simulink model "qbot2_sim_2019b"  (R2019b)
settings: Solver=FixedStepAuto  StartTime=0.0  StopTime=P.t_end  FixedStep=P.dt  RelTol=1e-3
InitFcn:
  | % load_qbot2_sim
StopFcn:
  | if (P.plotsim_flag)
  |     plot_sim(out, P)
  | end
(part 1 of 2)
settings Model: Creator=David L Olson  LastModifiedBy=divad

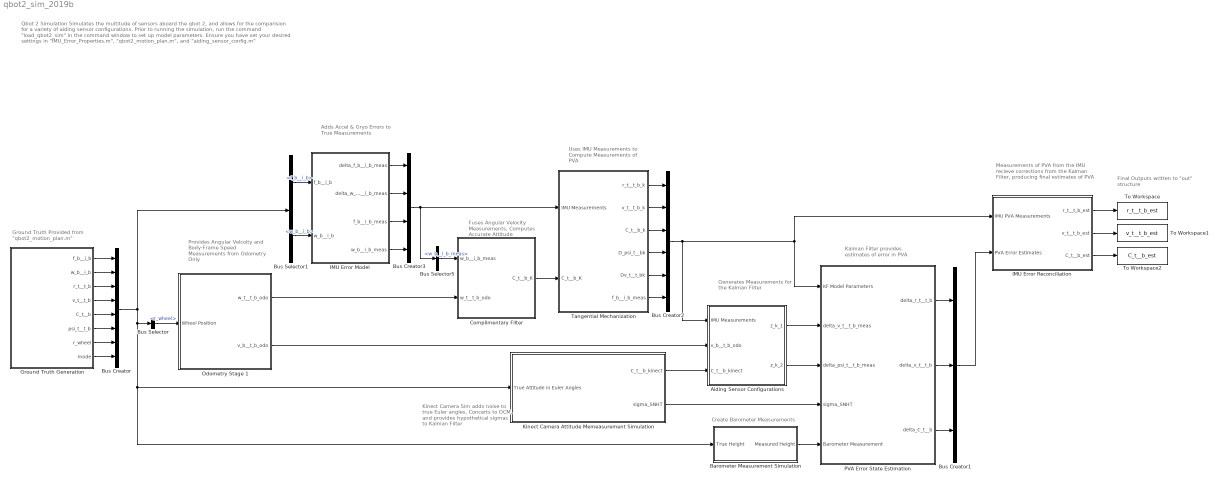
== system qbot2_sim_2019b ==
  note: Final Outputs written to "out" structure
  note: Create Barometer Measurements
  note: Qbot 2 Simulation
      |
      | Simulates the multitude of sensors aboard the qbot 2, and allows for the comparision for a variety of aiding sensor configurations.
      |
      | Prior to running the simulation, run the command "load_qbot2_sim" in the command window to set up model parameters.
      | Ensure you have set your desired settings in "IMU_Error_Properties.m", "qbot2_motion_plan.m", and "aiding_sensor_config.m"
  note: Measurements of PVA from the IMU recieve corrections from the Kalman Filter, producing final estimates of PVA
  note: Kalman Filter provides estimates of error in PVA
  note: Generates Measurements for the Kalman Filter
  note: Kinect Camera Sim adds noise to true Euler angles, Concerts to DCM, and provides hypothetical sigmas to Kalman Filter
  note: Uses IMU Measurements to Compute Measurements of PVA
  note: Fuses Angular Velocity Measurements, Computes Accurate Attitude
  note: Adds Accel & Gryo Errors to True Measurements
  note: Provides Angular Velcoity and Body-Frame Speed Measurements from Odometry Only
  note: Ground Truth Provided from "qbot2_motion_plan.m"
  Aiding Sensor Configurations : Subsystem
  Barometer Measurement Simulation : Subsystem
  Bus Creator : BusCreator  Inputs=8
  Bus Creator1 : BusCreator  Inputs=3
  Bus Creator2 : BusCreator  Inputs=6
  Bus Creator3 : BusCreator  Inputs=4
  Bus Selector : BusSelector  OutputSignals=r_wheel
  Bus Selector1 : BusSelector  OutputSignals=f_b__i_b,w_b__i_b
  Bus Selector5 : BusSelector  OutputSignals=w_b__i_b_meas
  Complimentary Filter : Subsystem
  Ground Truth Generation : Subsystem
  IMU Error Model : Subsystem
  IMU Error Reconciliation : Subsystem
  Kinect Camera Attitude Memeasurement Simulation : Subsystem
  Odometry Stage 1 : Subsystem
  PVA Error State Estimation : Subsystem
  Tangential Mechanization : Subsystem
  To Workspace : ToWorkspace  VariableName=r_t__t_b_est  SampleTime=-1
  To Workspace1 : ToWorkspace  VariableName=v_t__t_b_est  SampleTime=-1
  To Workspace2 : ToWorkspace  VariableName=C_t__b_est  SampleTime=-1
  wires:
  Ground Truth Generation/1(f_b__i_b) -> Bus Creator/1
  Ground Truth Generation/2(w_b__i_b) -> Bus Creator/2
  Ground Truth Generation/3(r_t__t_b) -> Bus Creator/3
  Ground Truth Generation/4(v_t__t_b) -> Bus Creator/4
  Ground Truth Generation/5(C_t__b) -> Bus Creator/5
  Bus Creator/1 -> Bus Selector1/1, Barometer Measurement Simulation/1(True Height), Kinect Camera Attitude Memeasurement Simulation/1(True Attitude in Euler Angles), Bus Selector/1
  Bus Selector/1 -> Odometry Stage 1/1(Wheel Position)  "<r_wheel>"
  Odometry Stage 1/1(w_t__t_b_odo) -> Complimentary Filter/2("w_t__t_b_odo ")
  Odometry Stage 1/2(v_b__t_b_odo) -> Aiding Sensor Configurations/2(v_b__t_b_odo)
  Aiding Sensor Configurations/1(z_k_1) -> PVA Error State Estimation/2(delta_v_t__t_b_meas)
  Aiding Sensor Configurations/2(z_k_2) -> PVA Error State Estimation/3(delta_psi_t__t_b_meas)
  Ground Truth Generation/6(psi_t__t_b) -> Bus Creator/6
  Ground Truth Generation/7(r_wheel) -> Bus Creator/7
  Ground Truth Generation/8(mode) -> Bus Creator/8
  Bus Selector1/1 -> IMU Error Model/1(f_b__i_b)  "<f_b__i_b>"
  Bus Selector1/2 -> IMU Error Model/2(w_b__i_b)  "<w_b__i_b>"
  Complimentary Filter/1(C_t__b_K) -> Tangential Mechanization/2("C_t__b_K ")
  Tangential Mechanization/1(r_t__t_b_k) -> Bus Creator2/1
  Tangential Mechanization/2(v_t__t_b_k) -> Bus Creator2/2
  Tangential Mechanization/3(C_t__b_k) -> Bus Creator2/3
  IMU Error Model/1(delta_f_b__i_b_meas) -> Bus Creator3/1
  IMU Error Model/2(delta_w_b__i_b_meas) -> Bus Creator3/2
  IMU Error Model/3(f_b__i_b_meas) -> Bus Creator3/3
  IMU Error Model/4(w_b__i_b_meas) -> Bus Creator3/4
  Bus Selector5/1 -> Complimentary Filter/1(w_b__i_b_meas)  "<w_b__i_b_meas>"
  Bus Creator3/1 -> Tangential Mechanization/1(IMU Measurements), Bus Selector5/1
  Tangential Mechanization/4(D_psi_t__bk) -> Bus Creator2/4
  Tangential Mechanization/5(Dv_t__t_bk) -> Bus Creator2/5
  Bus Creator2/1 -> IMU Error Reconciliation/1(IMU PVA Measurements), PVA Error State Estimation/1(KF Model Parameters), Aiding Sensor Configurations/1(IMU Measurements)
  Tangential Mechanization/6(f_b__i_b_meas) -> Bus Creator2/6
  PVA Error State Estimation/1(delta_r_t__t_b) -> Bus Creator1/1
  PVA Error State Estimation/2(delta_v_t__t_b) -> Bus Creator1/2
  PVA Error State Estimation/3(delta_C_t__b) -> Bus Creator1/3
  Barometer Measurement Simulation/1(Measured Height) -> PVA Error State Estimation/5(Barometer Measurement)
  Bus Creator1/1 -> IMU Error Reconciliation/2(PVA Error Estimates)
  IMU Error Reconciliation/1(r_t__t_b_est) -> To Workspace/1
  IMU Error Reconciliation/2(v_t__t_b_est) -> To Workspace1/1
  IMU Error Reconciliation/3(C_t__b_est) -> To Workspace2/1
  Kinect Camera Attitude Memeasurement Simulation/1(C_t__b_kinect) -> Aiding Sensor Configurations/3(C_t__b_kinect)
  Kinect Camera Attitude Memeasurement Simulation/2(sigma_SNHT) -> PVA Error State Estimation/4(sigma_SNHT)

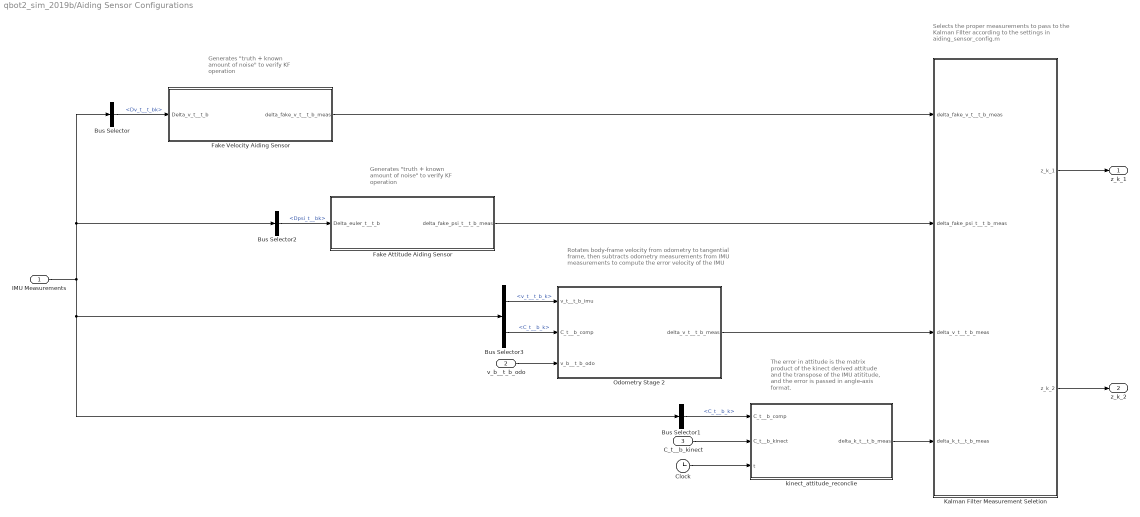
== system qbot2_sim_2019b/Aiding Sensor Configurations ==
  note: Selects the proper measurements to pass to the Kalman FIlter according to the settings in aiding_sensor_config.m
  note: The error in attitude is the matrix product of the kinect derived attitude and the transpose of the IMU atititude, and the error is passed in angle-axis format.
  note: Rotates body-frame velocity from odometry to tangential frame, then subtracts odometry measurements from IMU measurements to compute the error velocity of the IMU
  note: Generates "truth + known amount of noise" to verify KF operation
  note: Generates "truth + known amount of noise" to verify KF operation
  IMU Measurements : Inport
  v_b__t_b_odo : Inport  Port=2
  C_t__b_kinect : Inport  Port=3
  Bus Selector : BusSelector  OutputSignals=Dv_t__t_bk
  Bus Selector1 : BusSelector  OutputSignals=C_t__b_k
  Bus Selector2 : BusSelector  OutputSignals=Dpsi_t__bk
  Bus Selector3 : BusSelector  OutputSignals=v_t__t_b_k,C_t__b_k
  Clock : Clock
  Fake Attitude Aiding Sensor : MATLAB Function  TreatAsAtomicUnit=on
  Fake Velocity Aiding Sensor : MATLAB Function  TreatAsAtomicUnit=on
  Kalman Filter Measurement Seletion : MATLAB Function  TreatAsAtomicUnit=on
  Odometry Stage 2 : Subsystem
  kinect_attitude_reconclie : MATLAB Function  TreatAsAtomicUnit=on
  z_k_1 : Outport
  z_k_2 : Outport  Port=2
  wires:
  v_b__t_b_odo/1 -> Odometry Stage 2/3(v_b__t_b_odo)
  Fake Attitude Aiding Sensor/1(delta_fake_psi_t__t_b_meas) -> Kalman Filter Measurement Seletion/2(delta_fake_psi_t__t_b_meas)
  Fake Velocity Aiding Sensor/1(delta_fake_v_t__t_b_meas) -> Kalman Filter Measurement Seletion/1(delta_fake_v_t__t_b_meas)
  Odometry Stage 2/1(delta_v_t__t_b_meas) -> Kalman Filter Measurement Seletion/3(delta_v_t__t_b_meas)
  Kalman Filter Measurement Seletion/1(z_k_1) -> z_k_1/1
  Kalman Filter Measurement Seletion/2(z_k_2) -> z_k_2/1
  Bus Selector1/1 -> kinect_attitude_reconclie/1(C_t__b_comp)  "<C_t__b_k>"
  C_t__b_kinect/1 -> kinect_attitude_reconclie/2(C_t__b_kinect)
  kinect_attitude_reconclie/1(delta_k_t__t_b_meas) -> Kalman Filter Measurement Seletion/4(delta_k_t__t_b_meas)
  Bus Selector/1 -> Fake Velocity Aiding Sensor/1(Delta_v_t__t_b)  "<Dv_t__t_bk>"
  Bus Selector2/1 -> Fake Attitude Aiding Sensor/1(Delta_euler_t__t_b)  "<Dpsi_t__bk>"
  Bus Selector3/1 -> Odometry Stage 2/1(v_t__t_b_imu)  "<v_t__t_b_k>"
  Bus Selector3/2 -> Odometry Stage 2/2(C_t__b_comp)  "<C_t__b_k>"
  IMU Measurements/1 -> Bus Selector3/1, Bus Selector1/1, Bus Selector/1, Bus Selector2/1
  Clock/1 -> kinect_attitude_reconclie/3(t)

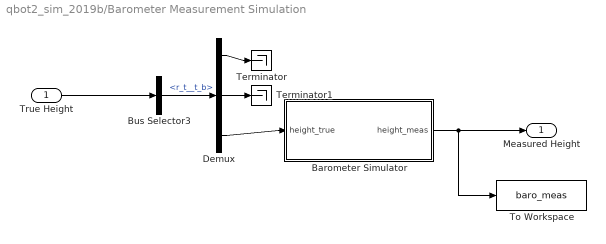
== system qbot2_sim_2019b/Barometer Measurement Simulation ==
  True Height : Inport
  Barometer Simulator : MATLAB Function  TreatAsAtomicUnit=on
  Bus Selector3 : BusSelector  OutputSignals=r_t__t_b
  Demux : Demux  Outputs=3
  Terminator : Terminator
  Terminator1 : Terminator
  To Workspace : ToWorkspace  VariableName=baro_meas  SampleTime=-1
  Measured Height : Outport
  wires:
  Demux/2 -> Terminator1/1
  True Height/1 -> Bus Selector3/1
  Bus Selector3/1 -> Demux/1  "<r_t__t_b>"
  Demux/3 -> Barometer Simulator/1(height_true)
  Demux/1 -> Terminator/1
  Barometer Simulator/1(height_meas) -> To Workspace/1, Measured Height/1

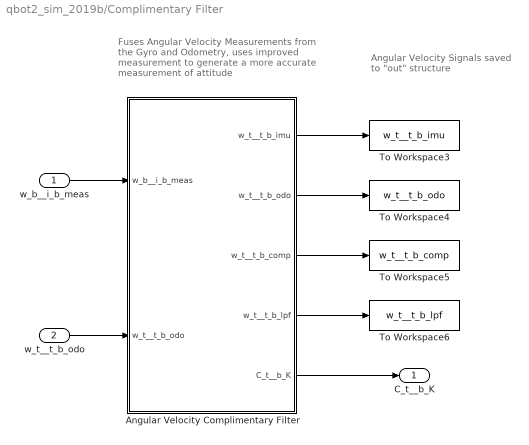
== system qbot2_sim_2019b/Complimentary Filter ==
  note: Fuses Angular Velocity Measurements from the Gyro and Odometry, uses improved measurement to generate a more accurate measurement of attitude
  note: Angular Velocity Signals saved to "out" structure
  w_b__i_b_meas : Inport
  "w_t__t_b_odo " : Inport  Port=2
  Angular Velocity Complimentary Filter : MATLAB Function  TreatAsAtomicUnit=on
  To Workspace3 : ToWorkspace  VariableName=w_t__t_b_imu  SampleTime=-1
  To Workspace4 : ToWorkspace  VariableName=w_t__t_b_odo  SampleTime=-1
  To Workspace5 : ToWorkspace  VariableName=w_t__t_b_comp  SampleTime=-1
  To Workspace6 : ToWorkspace  VariableName=w_t__t_b_lpf  SampleTime=-1
  C_t__b_K : Outport
  wires:
  Angular Velocity Complimentary Filter/4(w_t__t_b_lpf) -> To Workspace6/1
  w_b__i_b_meas/1 -> Angular Velocity Complimentary Filter/1(w_b__i_b_meas)
  "w_t__t_b_odo "/1 -> Angular Velocity Complimentary Filter/2("w_t__t_b_odo ")
  Angular Velocity Complimentary Filter/3(w_t__t_b_comp) -> To Workspace5/1
  Angular Velocity Complimentary Filter/2(w_t__t_b_odo) -> To Workspace4/1
  Angular Velocity Complimentary Filter/5(C_t__b_K) -> C_t__b_K/1
  Angular Velocity Complimentary Filter/1(w_t__t_b_imu) -> To Workspace3/1

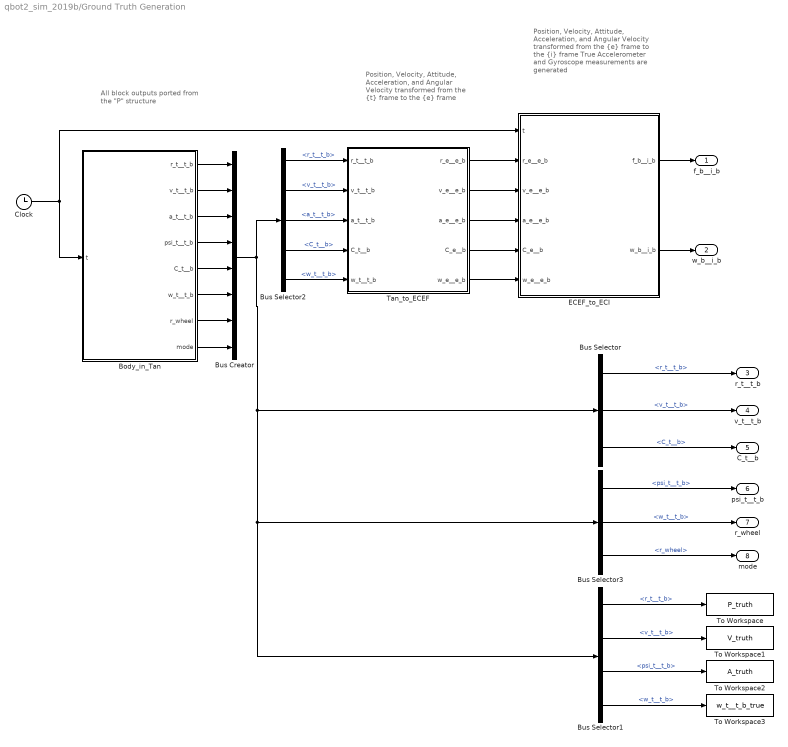
== system qbot2_sim_2019b/Ground Truth Generation ==
  note: Position, Velocity, Attitude, Acceleration, and Angular Velocity transformed from the {e} frame to the {i} frame
      |
      | True Accelerometer and Gyroscope measurements are generated
  note: Position, Velocity, Attitude, Acceleration, and Angular Velocity transformed from the {t} frame to the {e} frame
  note: All block outputs ported from the "P" structure
  Body_in_Tan : MATLAB Function  TreatAsAtomicUnit=on
  Bus Creator : BusCreator  Inputs=8
  Bus Selector : BusSelector  OutputSignals=r_t__t_b,v_t__t_b,C_t__b
  Bus Selector1 : BusSelector  OutputSignals=r_t__t_b,v_t__t_b,psi_t__t_b,w_t__t_b
  Bus Selector2 : BusSelector  OutputSignals=r_t__t_b,v_t__t_b,a_t__t_b,C_t__b,w_t__t_b
  Bus Selector3 : BusSelector  OutputSignals=psi_t__t_b,w_t__t_b,r_wheel
  Clock : Clock
  ECEF_to_ECI : MATLAB Function  TreatAsAtomicUnit=on
  Tan_to_ECEF : MATLAB Function  TreatAsAtomicUnit=on
  To Workspace : ToWorkspace  VariableName=P_truth  SampleTime=-1
  To Workspace1 : ToWorkspace  VariableName=V_truth  SampleTime=-1
  To Workspace2 : ToWorkspace  VariableName=A_truth  SampleTime=-1
  To Workspace3 : ToWorkspace  VariableName=w_t__t_b_true  SampleTime=-1
  f_b__i_b : Outport
  w_b__i_b : Outport  Port=2
  r_t__t_b : Outport  Port=3
  v_t__t_b : Outport  Port=4
  C_t__b : Outport  Port=5
  psi_t__t_b : Outport  Port=6
  r_wheel : Outport  Port=7
  mode : Outport  Port=8
  wires:
  Clock/1 -> ECEF_to_ECI/1(t), Body_in_Tan/1(t)
  Tan_to_ECEF/1(r_e__e_b) -> ECEF_to_ECI/2(r_e__e_b)
  Tan_to_ECEF/3(a_e__e_b) -> ECEF_to_ECI/4(a_e__e_b)
  Tan_to_ECEF/2(v_e__e_b) -> ECEF_to_ECI/3(v_e__e_b)
  Tan_to_ECEF/4(C_e__b) -> ECEF_to_ECI/5(C_e__b)
  Tan_to_ECEF/5(w_e__e_b) -> ECEF_to_ECI/6(w_e__e_b)
  ECEF_to_ECI/2(w_b__i_b) -> w_b__i_b/1
  ECEF_to_ECI/1(f_b__i_b) -> f_b__i_b/1
  Bus Selector/1 -> r_t__t_b/1  "<r_t__t_b>"
  Bus Selector/2 -> v_t__t_b/1  "<v_t__t_b>"
  Bus Selector/3 -> C_t__b/1  "<C_t__b>"
  Bus Selector2/5 -> Tan_to_ECEF/5(w_t__t_b)  "<w_t__t_b>"
  Bus Selector2/4 -> Tan_to_ECEF/4(C_t__b)  "<C_t__b>"
  Bus Selector2/3 -> Tan_to_ECEF/3(a_t__t_b)  "<a_t__t_b>"
  Bus Selector2/2 -> Tan_to_ECEF/2(v_t__t_b)  "<v_t__t_b>"
  Bus Selector2/1 -> Tan_to_ECEF/1(r_t__t_b)  "<r_t__t_b>"
  Bus Selector1/2 -> To Workspace1/1  "<v_t__t_b>"
  Bus Selector1/1 -> To Workspace/1  "<r_t__t_b>"
  Bus Selector1/3 -> To Workspace2/1  "<psi_t__t_b>"
  Bus Creator/1 -> Bus Selector2/1, Bus Selector/1, Bus Selector1/1, Bus Selector3/1
  Bus Selector3/2 -> r_wheel/1  "<w_t__t_b>"
  Bus Selector3/3 -> mode/1  "<r_wheel>"
  Body_in_Tan/1(r_t__t_b) -> Bus Creator/1
  Body_in_Tan/2(v_t__t_b) -> Bus Creator/2
  Body_in_Tan/3(a_t__t_b) -> Bus Creator/3
  Body_in_Tan/4(psi_t__t_b) -> Bus Creator/4
  Body_in_Tan/5(C_t__b) -> Bus Creator/5
  Body_in_Tan/6(w_t__t_b) -> Bus Creator/6
  Body_in_Tan/7(r_wheel) -> Bus Creator/7
  Body_in_Tan/8(mode) -> Bus Creator/8
  Bus Selector1/4 -> To Workspace3/1  "<w_t__t_b>"
  Bus Selector3/1 -> psi_t__t_b/1  "<psi_t__t_b>"

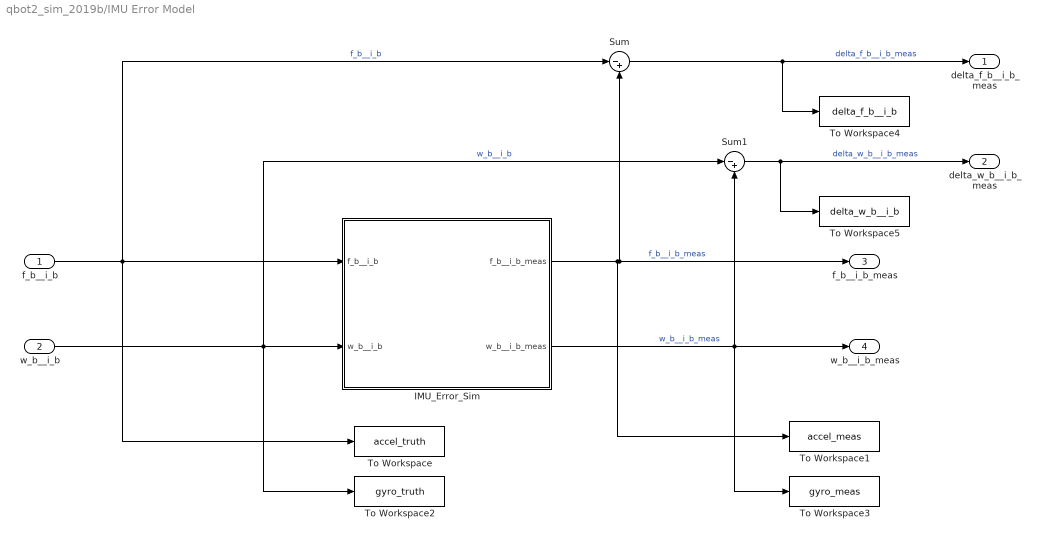
== system qbot2_sim_2019b/IMU Error Model ==
  f_b__i_b : Inport
  w_b__i_b : Inport  Port=2
  IMU_Error_Sim : MATLAB Function  TreatAsAtomicUnit=on
  Sum : Sum  Inputs=|-+
  Sum1 : Sum  Inputs=|-+
  To Workspace : ToWorkspace  VariableName=accel_truth  SampleTime=-1
  To Workspace1 : ToWorkspace  VariableName=accel_meas  SampleTime=-1
  To Workspace2 : ToWorkspace  VariableName=gyro_truth  SampleTime=-1
  To Workspace3 : ToWorkspace  VariableName=gyro_meas  SampleTime=-1
  To Workspace4 : ToWorkspace  VariableName=delta_f_b__i_b  SampleTime=-1
  To Workspace5 : ToWorkspace  VariableName=delta_w_b__i_b  SampleTime=-1
  delta_f_b__i_b_meas : Outport
  delta_w_b__i_b_meas : Outport  Port=2
  f_b__i_b_meas : Outport  Port=3
  w_b__i_b_meas : Outport  Port=4
  wires:
  f_b__i_b/1 -> To Workspace/1, Sum/1, IMU_Error_Sim/1(f_b__i_b)  "f_b__i_b"
  w_b__i_b/1 -> Sum1/1, To Workspace2/1, IMU_Error_Sim/2(w_b__i_b)  "w_b__i_b"
  IMU_Error_Sim/1(f_b__i_b_meas) -> f_b__i_b_meas/1, Sum/2, To Workspace1/1  "f_b__i_b_meas"
  IMU_Error_Sim/2(w_b__i_b_meas) -> Sum1/2, w_b__i_b_meas/1, To Workspace3/1  "w_b__i_b_meas"
  Sum1/1 -> To Workspace5/1, delta_w_b__i_b_meas/1  "delta_w_b__i_b_meas"
  Sum/1 -> To Workspace4/1, delta_f_b__i_b_meas/1  "delta_f_b__i_b_meas"

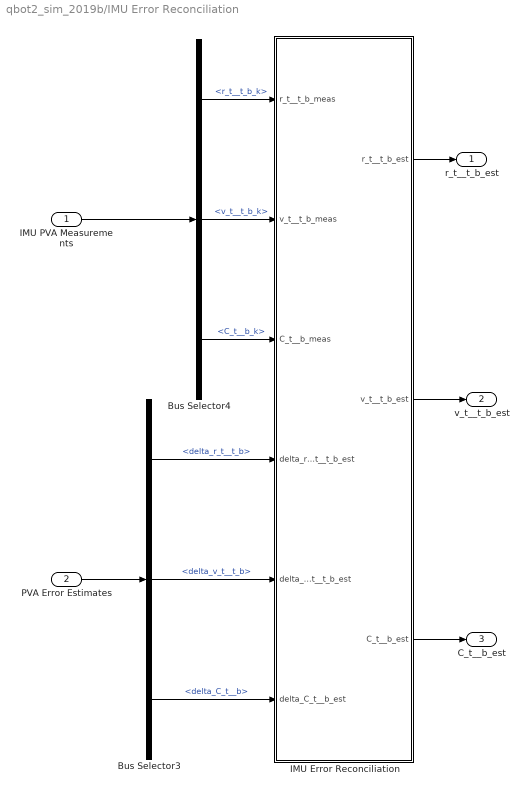
== system qbot2_sim_2019b/IMU Error Reconciliation ==
  IMU PVA Measurements : Inport
  PVA Error Estimates : Inport  Port=2
  Bus Selector3 : BusSelector  OutputSignals=delta_r_t__t_b,delta_v_t__t_b,delta_C_t__b
  Bus Selector4 : BusSelector  OutputSignals=r_t__t_b_k,v_t__t_b_k,C_t__b_k
  IMU Error Reconciliation : MATLAB Function  TreatAsAtomicUnit=on
  r_t__t_b_est : Outport
  v_t__t_b_est : Outport  Port=2
  C_t__b_est : Outport  Port=3
  wires:
  Bus Selector3/1 -> IMU Error Reconciliation/4(delta_r_t__t_b_est)  "<delta_r_t__t_b>"
  IMU Error Reconciliation/3(C_t__b_est) -> C_t__b_est/1
  Bus Selector4/2 -> IMU Error Reconciliation/2(v_t__t_b_meas)  "<v_t__t_b_k>"
  Bus Selector4/3 -> IMU Error Reconciliation/3(C_t__b_meas)  "<C_t__b_k>"
  IMU PVA Measurements/1 -> Bus Selector4/1
  Bus Selector3/2 -> IMU Error Reconciliation/5(delta_v_t__t_b_est)  "<delta_v_t__t_b>"
  IMU Error Reconciliation/2(v_t__t_b_est) -> v_t__t_b_est/1
  Bus Selector4/1 -> IMU Error Reconciliation/1(r_t__t_b_meas)  "<r_t__t_b_k>"
  Bus Selector3/3 -> IMU Error Reconciliation/6(delta_C_t__b_est)  "<delta_C_t__b>"
  PVA Error Estimates/1 -> Bus Selector3/1
  IMU Error Reconciliation/1(r_t__t_b_est) -> r_t__t_b_est/1

== system qbot2_sim_2019b/Kinect Camera Attitude Memeasurement Simulation ==
  True Attitude in Euler Angles : Inport
  Bus Selector2 : BusSelector  OutputSignals=psi_t__t_b
  Clock : Clock
  Kinect Camera Sim : MATLAB Function  TreatAsAtomicUnit=on
  C_t__b_kinect : Outport
  sigma_SNHT : Outport  Port=2
  wires:
  Kinect Camera Sim/2(sigma_SNHT) -> sigma_SNHT/1
  Kinect Camera Sim/1(C_t__b_kinect) -> C_t__b_kinect/1
  Bus Selector2/1 -> Kinect Camera Sim/2(psi_t__t_b)  "<psi_t__t_b>"
  Clock/1 -> Kinect Camera Sim/1(t)
  True Attitude in Euler Angles/1 -> Bus Selector2/1

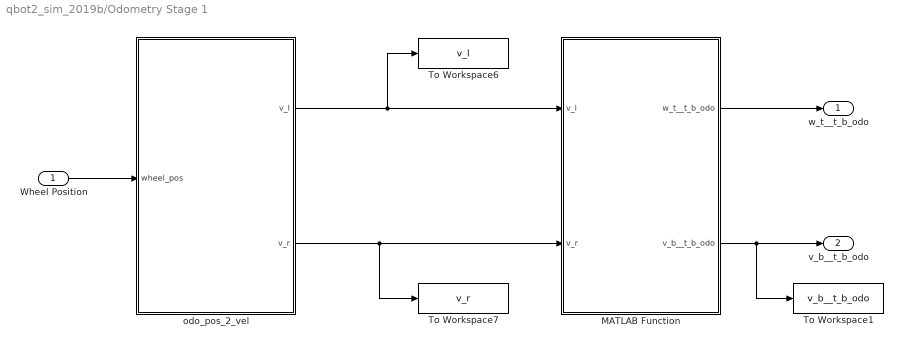
== system qbot2_sim_2019b/Odometry Stage 1 ==
  Wheel Position : Inport
  MATLAB Function : MATLAB Function  TreatAsAtomicUnit=on
  To Workspace1 : ToWorkspace  VariableName=v_b__t_b_odo  SampleTime=-1
  To Workspace6 : ToWorkspace  VariableName=v_l  SampleTime=-1
  To Workspace7 : ToWorkspace  VariableName=v_r  SampleTime=-1
  odo_pos_2_vel : MATLAB Function  TreatAsAtomicUnit=on
  w_t__t_b_odo : Outport
  v_b__t_b_odo : Outport  Port=2
  wires:
  Wheel Position/1 -> odo_pos_2_vel/1(wheel_pos)
  MATLAB Function/1(w_t__t_b_odo) -> w_t__t_b_odo/1
  odo_pos_2_vel/1(v_l) -> To Workspace6/1, MATLAB Function/1(v_l)
  odo_pos_2_vel/2(v_r) -> To Workspace7/1, MATLAB Function/2(v_r)
  MATLAB Function/2(v_b__t_b_odo) -> To Workspace1/1, v_b__t_b_odo/1

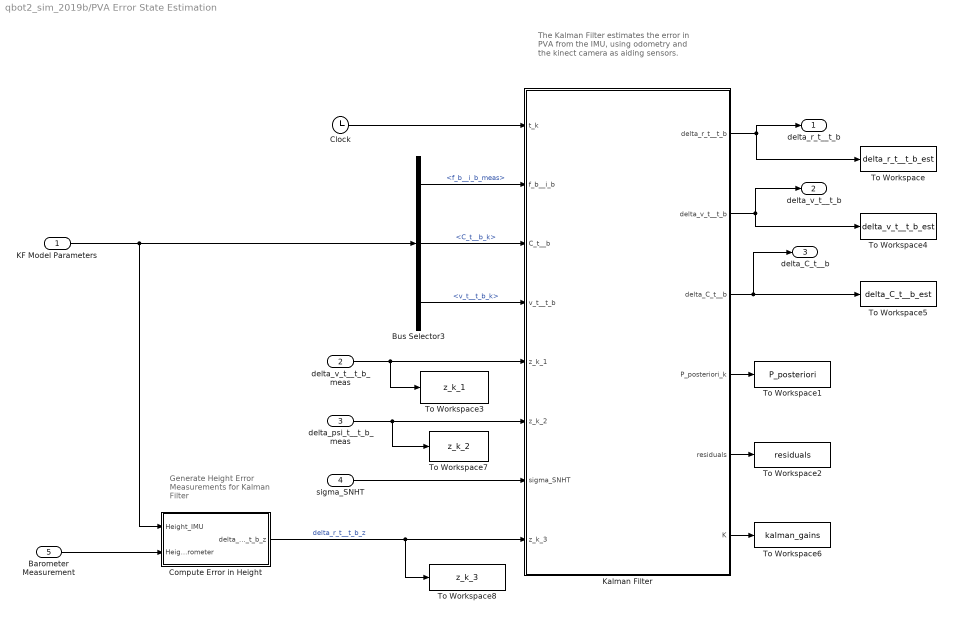
== system qbot2_sim_2019b/PVA Error State Estimation ==
  note: Generate Height Error Measurements for Kalman Filter
  note: The Kalman Filter estimates the error in PVA from the IMU, using odometry and the kinect camera as aiding sensors.
  KF Model Parameters : Inport
  delta_v_t__t_b_meas : Inport  Port=2
  delta_psi_t__t_b_meas : Inport  Port=3
  sigma_SNHT : Inport  Port=4
  Barometer Measurement : Inport  Port=5
  Bus Selector3 : BusSelector  OutputSignals=f_b__i_b_meas,C_t__b_k,v_t__t_b_k
  Clock : Clock
  Compute Error in Height : Subsystem
  Kalman Filter : MATLAB Function  TreatAsAtomicUnit=on
  To Workspace : ToWorkspace  VariableName=delta_r_t__t_b_est  SampleTime=-1
  To Workspace1 : ToWorkspace  VariableName=P_posteriori  SampleTime=-1
  To Workspace2 : ToWorkspace  VariableName=residuals  SampleTime=-1
  To Workspace3 : ToWorkspace  VariableName=z_k_1  SampleTime=-1
  To Workspace4 : ToWorkspace  VariableName=delta_v_t__t_b_est  SampleTime=-1
  To Workspace5 : ToWorkspace  VariableName=delta_C_t__b_est  SampleTime=-1
  To Workspace6 : ToWorkspace  VariableName=kalman_gains  SampleTime=-1
  To Workspace7 : ToWorkspace  VariableName=z_k_2  SampleTime=-1
  To Workspace8 : ToWorkspace  VariableName=z_k_3  SampleTime=-1
  delta_r_t__t_b : Outport
  delta_v_t__t_b : Outport  Port=2
  delta_C_t__b : Outport  Port=3
  wires:
  Kalman Filter/4(P_posteriori_k) -> To Workspace1/1
  Kalman Filter/5(residuals) -> To Workspace2/1
  Kalman Filter/1(delta_r_t__t_b) -> delta_r_t__t_b/1, To Workspace/1
  Kalman Filter/2(delta_v_t__t_b) -> delta_v_t__t_b/1, To Workspace4/1
  Kalman Filter/3(delta_C_t__b) -> delta_C_t__b/1, To Workspace5/1
  Kalman Filter/6(K) -> To Workspace6/1
  Bus Selector3/1 -> Kalman Filter/2(f_b__i_b)  "<f_b__i_b_meas>"
  Bus Selector3/2 -> Kalman Filter/3(C_t__b)  "<C_t__b_k>"
  Bus Selector3/3 -> Kalman Filter/4(v_t__t_b)  "<v_t__t_b_k>"
  delta_psi_t__t_b_meas/1 -> To Workspace7/1, Kalman Filter/6(z_k_2)
  delta_v_t__t_b_meas/1 -> To Workspace3/1, Kalman Filter/5(z_k_1)
  Clock/1 -> Kalman Filter/1(t_k)
  sigma_SNHT/1 -> Kalman Filter/7(sigma_SNHT)
  KF Model Parameters/1 -> Compute Error in Height/1(Height_IMU), Bus Selector3/1
  Barometer Measurement/1 -> Compute Error in Height/2(Height_Barometer)
  Compute Error in Height/1(delta_r_t__t_b_z) -> To Workspace8/1, Kalman Filter/8(z_k_3)  "delta_r_t__t_b_z"

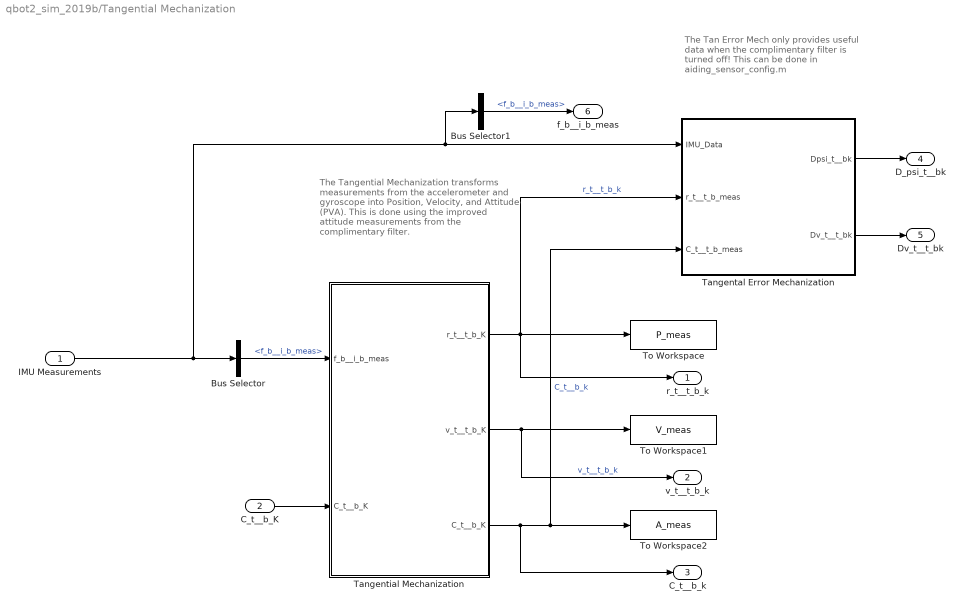
== system qbot2_sim_2019b/Tangential Mechanization ==
  note: The Tan Error Mech only provides useful data when the complimentary filter is turned off!
      |
      | This can be done in aiding_sensor_config.m
  note: The Tangential Mechanization transforms measurements from the accelerometer and gyroscope into Position, Velocity, and Attitude (PVA). This is done using the improved attitude measurements from the complimentary filter.
  IMU Measurements : Inport
  "C_t__b_K " : Inport  Port=2
  Bus Selector : BusSelector  OutputSignals=f_b__i_b_meas
  Bus Selector1 : BusSelector  OutputSignals=f_b__i_b_meas
  Tangental Error Mechanization : Subsystem
  Tangential Mechanization : MATLAB Function  TreatAsAtomicUnit=on
  To Workspace : ToWorkspace  VariableName=P_meas  SampleTime=-1
  To Workspace1 : ToWorkspace  VariableName=V_meas  SampleTime=-1
  To Workspace2 : ToWorkspace  VariableName=A_meas  SampleTime=-1
  r_t__t_b_k : Outport
  v_t__t_b_k : Outport  Port=2
  C_t__b_k : Outport  Port=3
  D_psi_t__bk : Outport  Port=4
  Dv_t__t_bk : Outport  Port=5
  f_b__i_b_meas : Outport  Port=6
  wires:
  Tangential Mechanization/1(r_t__t_b_K) -> Tangental Error Mechanization/2(r_t__t_b_meas), r_t__t_b_k/1, To Workspace/1  "r_t__t_b_k"
  Tangential Mechanization/2(v_t__t_b_K) -> v_t__t_b_k/1, To Workspace1/1  "v_t__t_b_k"
  Tangential Mechanization/3(C_t__b_K) -> C_t__b_k/1, Tangental Error Mechanization/3(C_t__t_b_meas), To Workspace2/1  "C_t__b_k"
  "C_t__b_K "/1 -> Tangential Mechanization/2("C_t__b_K ")
  IMU Measurements/1 -> Bus Selector1/1, Tangental Error Mechanization/1(IMU_Data), Bus Selector/1
  Bus Selector/1 -> Tangential Mechanization/1(f_b__i_b_meas)  "<f_b__i_b_meas>"
  Tangental Error Mechanization/1(Dpsi_t__bk) -> D_psi_t__bk/1
  Tangental Error Mechanization/2(Dv_t__t_bk) -> Dv_t__t_bk/1
  Bus Selector1/1 -> f_b__i_b_meas/1  "<f_b__i_b_meas>"

== system qbot2_sim_2019b/Aiding Sensor Configurations/Odometry Stage 2 ==
  v_t__t_b_imu : Inport
  C_t__b_comp : Inport  Port=2
  v_b__t_b_odo : Inport  Port=3
  Rotate_Speed : MATLAB Function  TreatAsAtomicUnit=on
  Sum : Sum  Inputs=-+|
  To Workspace3 : ToWorkspace  VariableName=v_t__t_b_odo  SampleTime=-1
  delta_v_t__t_b_meas : Outport
  wires:
  Rotate_Speed/1(v_t__t_b_odo) -> To Workspace3/1, Sum/2  "v_t__t_b_odo"
  Sum/1 -> delta_v_t__t_b_meas/1  "delta_v_t__t_b_meas"
  v_b__t_b_odo/1 -> Rotate_Speed/2(v_b__t_b_odo)
  v_t__t_b_imu/1 -> Sum/1
  C_t__b_comp/1 -> Rotate_Speed/1(C_t__b_k)

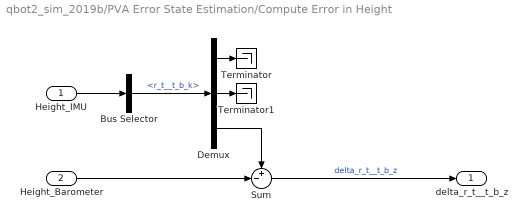
== system qbot2_sim_2019b/PVA Error State Estimation/Compute Error in Height ==
  Height_IMU : Inport
  Height_Barometer : Inport  Port=2
  Bus Selector : BusSelector  OutputSignals=r_t__t_b_k
  Demux : Demux  Outputs=3
  Sum : Sum  Inputs=+-|
  Terminator : Terminator
  Terminator1 : Terminator
  delta_r_t__t_b_z : Outport
  wires:
  Demux/3 -> Sum/1
  Demux/1 -> Terminator/1
  Demux/2 -> Terminator1/1
  Bus Selector/1 -> Demux/1  "<r_t__t_b_k>"
  Sum/1 -> delta_r_t__t_b_z/1  "delta_r_t__t_b_z"
  Height_Barometer/1 -> Sum/2
  Height_IMU/1 -> Bus Selector/1

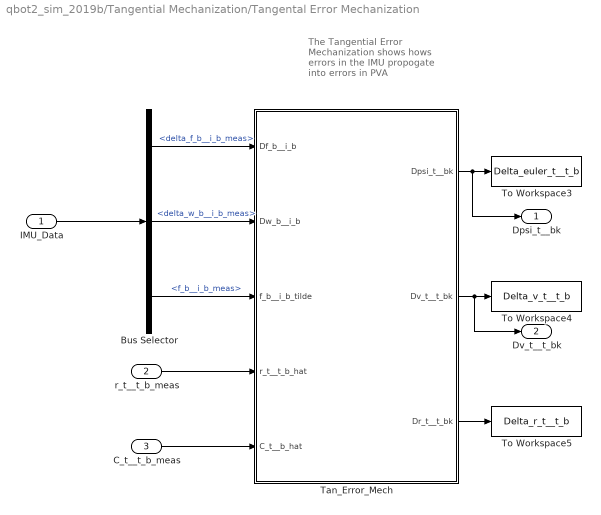
== system qbot2_sim_2019b/Tangential Mechanization/Tangental Error Mechanization ==
  note: The Tangential Error Mechanization shows hows errors in the IMU propogate into errors in PVA
  IMU_Data : Inport
  r_t__t_b_meas : Inport  Port=2
  C_t__t_b_meas : Inport  Port=3
  Bus Selector : BusSelector  OutputSignals=delta_f_b__i_b_meas,delta_w_b__i_b_meas,f_b__i_b_meas
  Tan_Error_Mech : MATLAB Function  TreatAsAtomicUnit=on
  To Workspace3 : ToWorkspace  VariableName=Delta_euler_t__t_b  SampleTime=-1
  To Workspace4 : ToWorkspace  VariableName=Delta_v_t__t_b  SampleTime=-1
  To Workspace5 : ToWorkspace  VariableName=Delta_r_t__t_b  SampleTime=-1
  Dpsi_t__bk : Outport
  Dv_t__t_bk : Outport  Port=2
  wires:
  Tan_Error_Mech/1(Dpsi_t__bk) -> Dpsi_t__bk/1, To Workspace3/1
  Tan_Error_Mech/2(Dv_t__t_bk) -> Dv_t__t_bk/1, To Workspace4/1
  Tan_Error_Mech/3(Dr_t__t_bk) -> To Workspace5/1
  IMU_Data/1 -> Bus Selector/1
  Bus Selector/1 -> Tan_Error_Mech/1(Df_b__i_b)  "<delta_f_b__i_b_meas>"
  Bus Selector/2 -> Tan_Error_Mech/2(Dw_b__i_b)  "<delta_w_b__i_b_meas>"
  Bus Selector/3 -> Tan_Error_Mech/3(f_b__i_b_tilde)  "<f_b__i_b_meas>"
  r_t__t_b_meas/1 -> Tan_Error_Mech/4(r_t__t_b_hat)
  C_t__t_b_meas/1 -> Tan_Error_Mech/5(C_t__b_hat)

== matlab function qbot2_sim_2019b/Ground Truth Generation/Body_in_Tan ==
  data: r_t__t_b output; v_t__t_b output; a_t__t_b output; psi_t__t_b output; C_t__b output; w_t__t_b output; t input; P parameter; r_wheel output; mode output
function [r_t__t_b, v_t__t_b, a_t__t_b, psi_t__t_b, C_t__b, w_t__t_b, r_wheel, mode] = ...
                                           Body_in_Tan(t, P)
                                       
%% QBOT2_TAN_GROUND_TRUTH_GEN Generates the motion of the body of the Qbot2
%wrt to the tangential frame.  

% Creating figure eight loop pattern for Qbot2.  The motion is unrealistic
% for the robot itself, however for now this verify all equations have been
% implemented correctly in all 3 dimensions.  

persistent k

% Initialize k on first run
if (isempty(k))
    k = 1;
end

% Pull Motion Plan Values from P structure
r_t__t_b = P.r_t__t_b(:,k);
v_t__t_b = P.v_t__t_b(:,k);
a_t__t_b = P.a_t__t_b(:,k);
psi_t__t_b = [0; 0; P.psi_t__t_b(k)];
C_t__b = rotate_z(psi_t__t_b(3));
w_t__t_b = P.w_t__t_b(:,k);
r_wheel = P.r_wheel(:,k);
mode = P.mode(k);

% Normalize C_t__b
C_t__b = q2dcm(dcm2q(C_t__b));

% Update k
k = k + 1;

end

== matlab function qbot2_sim_2019b/Tangential Mechanization/Tangential Mechanization ==
  data: f_b__i_b_meas input; C_t__b_K input; r_t__t_b_K output; P parameter; v_t__t_b_K output; C_t__b_K output
function [r_t__t_b_K, v_t__t_b_K, C_t__b_K] = Tan_Mech(f_b__i_b_meas, C_t__b_K, P)

%% Tan_Mech
% Provides tangential mechanization for kinematic states position, velocity
% and attitude (PVA).  It does this solely based on accel and gyro
% measurements, which come from the IMU block.  The first time step is
% initialized from the ground truth block.  

persistent r_t__t_b_K_1 v_t__t_b_K_1 g_t__b

% Initialize on First Time Step
if (isempty(r_t__t_b_K_1))
    
    % Use "truth" to initialize on first time step
    r_t__t_b_K = [0; 0; 0];
    v_t__t_b_K = [0; 0; 0];
    
    % Store current values as old values for next iteration
    r_t__t_b_K_1 = r_t__t_b_K;
    v_t__t_b_K_1 = v_t__t_b_K;
    
    % Calculate and store the vector g_t__b
    r_e__e_b = P.r_e__e_t + P.C_e__t*r_t__t_b_K;         % Compute r_e__e_b
    [L_b, lambda_b, h_b] = xyz2llh(r_e__e_b, P);            % Compute the lat, lon, and height
    g_n__b = [0; 0; gravity(L_b, h_b, P)];                  % Compute the acceleration due to gravity
    C_e__n = Lat_Lon_2C_e__n(L_b, lambda_b);                % Compute C_e__n
    g_e__b = C_e__n * g_n__b;                               % Compute the gravity of the body in the {e} frame
    g_t__b = P.C_e__t' * g_e__b;                            % Compute the gravity of the body in the {t} frame 
    
% Every Other Time Step____________________________________________________
else
    
    % f_t__i_b Specific Force Update
    f_t__i_b = C_t__b_K * f_b__i_b_meas;
    
    % a_t__t_b Acceleration Vector Update
    
    a_t__t_b = f_t__i_b + g_t__b - 2*P.Ohm_t__i_e*v_t__t_b_K_1;
    
    % v_t__t_b Velocity Vector Update
    v_t__t_b_K = v_t__t_b_K_1 + a_t__t_b*P.dt;
    
    % r_t__t_b Position Vector Update
    r_t__t_b_K = r_t__t_b_K_1 + v_t__t_b_K_1*P.dt + a_t__t_b*((P.dt^2)/2);
    
    % Store new PVA as old PVA
    r_t__t_b_K_1 = r_t__t_b_K;
    v_t__t_b_K_1 = v_t__t_b_K;
    
end

== matlab function qbot2_sim_2019b/Ground Truth Generation/Tan_to_ECEF ==
  data: r_t__t_b input; v_t__t_b input; a_t__t_b input; C_t__b input; w_t__t_b input; r_e__e_b output; v_e__e_b output; a_e__e_b output; C_e__b output; w_e__e_b output; P parameter
function [r_e__e_b, v_e__e_b, a_e__e_b, C_e__b, w_e__e_b] = ...
             Tan_to_ECEF(r_t__t_b, v_t__t_b, a_t__t_b, C_t__b, w_t__t_b, P)
         
%% Tan_to_ECEF 
% Transfroms motion in the {t} frame into the {e} frame.  The 'P' structure
% contains data relevant to making the {t}->{e} transforms specifically to
% my house in Minot ND.  (1124 9th St NW, Minot ND 58703)

% Position of the {b} frame wrt the {e} frame resolved in {e} (m)
r_e__e_b = P.r_e__e_t + P.C_e__t*r_t__t_b;

% Velocity of the {b} frame wrt the {e} frame resolved in {e} (m/s)
v_e__e_b = P.C_e__t*v_t__t_b;
       
% Acceleration of the b-frame wrt the e-frame resolved in {e} (m/s^2)
a_e__e_b = P.C_e__t*a_t__t_b;
        
%Attitude of the {b} frame wrt the {e} frame (unitless)
C_e__b = P.C_e__t*C_t__b;         

% Normalize C_e__b
C_e__b = q2dcm(dcm2q(C_e__b));

% Angular velocity of the {b} frame wrt the {e} frame resolved in {e} (rad/s)
w_e__e_b = P.C_e__t*w_t__t_b;

== matlab function qbot2_sim_2019b/Ground Truth Generation/ECEF_to_ECI ==
  data: t input; f_b__i_b output; r_e__e_b input; v_e__e_b input; a_e__e_b input; C_e__b input; w_e__e_b input; w_b__i_b output; P parameter
function [f_b__i_b, w_b__i_b] = ...
          ECEF_to_ECI(t, r_e__e_b, v_e__e_b, a_e__e_b, C_e__b, w_e__e_b, P)

%% ECEF to ECI
% Transforms motion from the ECEF frame to the ECI frame
% This assumes the simulation always starts at 0000z

% Calculate g_n__b only once, since area of travel is so small
persistent g_e__b

if (isempty(g_e__b))
    [L_b, lambda_b, h_b] = xyz2llh(r_e__e_b, P);
    g_n__b = [0; 0; gravity(L_b, h_b, P)];
    C_e__n = Lat_Lon_2C_e__n(L_b, lambda_b);
    g_e__b = C_e__n * g_n__b;
end

% Generate earth's rotation from {i} frame to {e} frame
theta_ie = P.w_ie * t + 0;

C_i__e = [cos(theta_ie), -sin(theta_ie), 0; ...
          sin(theta_ie),  cos(theta_ie), 0; ...
          0,              0,             1];    
      
% Position of {b} frame wrt {t} frame resolved in {i} frame (m)
r_i__i_b = C_i__e*r_e__e_b;

% Velocity of {b} frame wrt {i} frame resolved in {i} frame (m/s)
v_i__i_b = C_i__e*v_e__e_b + P.Ohm_i__i_e*C_i__e*r_e__e_b;

% Acceleration of {b} frame wrt {i} frame resolved in {i} frame (m/s^2)
a_i__i_b = C_i__e*a_e__e_b + 2*P.Ohm_i__i_e*C_i__e*v_e__e_b + ...
                                 P.Ohm_i__i_e*P.Ohm_i__i_e*C_i__e*r_e__e_b;
                                       
% Attitude of {b} frame wrt to {i} frame
C_i__b = C_i__e*C_e__b;

% Normalize C_i__b
C_i__b = q2dcm(dcm2q(C_i__b));

% Angular Velocity: Ideal Gyro Measurements
w_b__i_b = C_i__b' * (P.w_i__i_e + C_i__e*w_e__e_b);

% Specific Force: Ideal Accel Measurements
f_b__i_b = C_i__b' * (a_i__i_b - C_i__e*g_e__b - ...
                                       P.Ohm_i__i_e*P.Ohm_i__i_e*r_i__i_b);

== matlab function qbot2_sim_2019b/IMU Error Model/IMU_Error_Sim ==
  data: f_b__i_b input; f_b__i_b_meas output; w_b__i_b input; w_b__i_b_meas output; P parameter
function [f_b__i_b_meas, w_b__i_b_meas] = IMU(f_b__i_b, w_b__i_b, P)
% IMU models the IMU error characteristics, taking truth as the input and
% outputs measurements that are subject to errors.  These errors stem from
% data obtained from the VN200 used for hardware implementation.  

%% Function Initializatoin

persistent b_g_BI b_a_BI

if isempty(b_g_BI)
    b_g_BI = [0; 0; 0];
    b_a_BI = [0; 0; 0];
end

%% Define P

%  General P
dt = P.dt;
Fs = P.Fs;
I3 = eye(3);

% Gyro Related Terms
b_g_BI_sigma_n = P.gyro.BI.sigma_n;  % Bias - White Noise driving the Bias Instability 1-sigma (rad/s)

tau_g        = P.gyro.BI.correlation_time;  % Correlation time for the bias instability (sec)
b_g_FB       = P.gyro.b_g_FB;               % Bias - Fixed Bias term (rad/s)

sigma_ARW   = P.gyro.sigma_ARW;             % Standard deviation of white noise due to ARW (rad/s)
M_g         = P.gyro.M_g;                   % The combined Gyro Misalignment/Scale-Factor matrix
G_g         = P.gyro.G_g;                   % The gyro G-sensitivity matrix (rad/sec/g)

 % Accel related terms   
b_a_BI_sigma_n = P.accel.BI.sigma_n;        % Bias - White noise driving the Bias Instability 1-sigma (m/s^2)

tau_a        = P.accel.BI.correlation_time; % Correlation time for the bias instability (sec)
b_a_FB       = P.accel.b_a_FB;              % Bias - Fixed Bias term (m/s^2)

sigma_VRW   = P.accel.sigma_VRW;            % Standard deviation of white noise due to VRW (m/s^2)
M_a         = P.accel.M_a;                  % The combined Gyro Misalignment/Scale-Factor matrix    

% Build randn quantities from etrinsic functions
coder.extrinsic('randn');

% Preallocate Memory
randn1 = zeros(3,1);
randn2 = zeros(3,1);
randn3 = zeros(3,1);
randn4 = zeros(3,1);

% Build the randn variables
randn1 = randn(3,1);
randn2 = randn(3,1);
randn3 = randn(3,1);
randn4 = randn(3,1);

%++++++++++++++++++++++++++++++++++++++++++++++++++++++++++++++++++++++++++
% Gyro Model:
%++++++++++++++++++++++++++++++++++++++++++++++++++++++++++++++++++++++++++

% Bias terms
b_g_BS = P.gyro.b_g_BS;                                        % Bias - Bias Stability Bias term (rad/s)
b_g_BI = exp(-dt/tau_g) * b_g_BI + randn1.*b_g_BI_sigma_n; % Bias - Markov Bias Instability Bias term (rad/s)
b_g = b_g_BI + b_g_FB + b_g_BS;                                % All three bias terms (rad/s)

% Noise terms
w_g = sigma_ARW .* randn2;                                 % Gyro noise (rad/sec)

% Including all of the error terms
w_b__i_b_meas = b_g + (I3 + M_g) * w_b__i_b + G_g * f_b__i_b + w_g;

%++++++++++++++++++++++++++++++++++++++++++++++++++++++++++++++++++++++++++
% Accelerometer Model
%++++++++++++++++++++++++++++++++++++++++++++++++++++++++++++++++++++++++++

% Bias terms
b_a_BS = P.accel.b_a_BS;                                       % Bias - Bias Stability Bias term (m/s^2)
b_a_BI = exp(-dt/tau_a) * b_a_BI + randn3.*b_a_BI_sigma_n; % Bias - Markov Bias Instability Bias term (m/s^2)
b_a = b_a_BI + b_a_FB + b_a_BS;                                % All three bias terms (m/s^2)

% Noise terms
w_a = sigma_VRW .* randn4;                                 % Accelerometer noise (in m/s^2)

% Including all of the error terms
f_b__i_b_meas = b_a + (I3 + M_a) * f_b__i_b + w_a;

== matlab function qbot2_sim_2019b/Tangential Mechanization/Tangental Error Mechanization/Tan_Error_Mech ==
  data: Df_b__i_b input; Dpsi_t__bk output; Dw_b__i_b input; f_b__i_b_tilde input; r_t__t_b_hat input; C_t__b_hat input; Dv_t__t_bk output; Dr_t__t_bk output; P parameter
function [Dpsi_t__bk, Dv_t__t_bk, Dr_t__t_bk] = Tan_Error_mech(Df_b__i_b, Dw_b__i_b, f_b__i_b_tilde, r_t__t_b_hat, C_t__b_hat, P)
%#codegen
% FUNCTION DESCRIPTION:
%   Implements the Tangential Frame Error-Mechanization
%
% INPUTS:
%   Df_b__i_b       = Error in Current Accel measurements (m/s^2)
%   Dw_b__i_b       = Error in Current gyro measurements (rad/s)
%   f_b__i_b_tilde  = Current Accel measurements (m/s^2)
%   r_t__t_b_hat    = Position estimate from TAN mech (meters)
%   C_t__b_hat      = Attitude estimate from TAN mech
%
% OUTPUTS:
%   Dpsi_t__bk      = Delta psi      vector (rad)
%   Dv_t__t_bk      = Delta velocity vector (meters/sec)
%   Dr_t__t_bk      = Delta position vector (meters)
%
%  Reference:  EE 440 Lecture notes:
%       lectures 29 & 30
%  NOTES:
%    Groves Chap 14 Section 2

persistent Delta_PVAk_1

dt         = P.dt;          % Time step (sec)
I3         = eye(3);                % 3X3 Identity matrix
Ohm_i__i_e = P.Ohm_i__i_e;  % Skew symmetric version of w_i__i_e (rad/s)
C_e__t     = P.C_e__t;   	% Attitude of t-frame wrt e-frame (a constant matrix)
C_t__e     = C_e__t';
r_e__e_t   = P.r_e__e_t;    % Position of org of t-frame wrt e-frame resolved in e-frame
   
if isempty(Delta_PVAk_1)    
    Delta_PVAk_1  = zeros(9,1);     % Initialize Delta_PVA(k-1)
    Delta_PVAk    = zeros(9,1);     % Initialize Delta_PVA(k-1)
else
    Delta_PVAk = eye(9);
%% Build the F matrix: See lecture 29 slide 7
    O3 = zeros(3,3);
% First row:
    Ohm_t__i_e = C_t__e * Ohm_i__i_e * C_e__t;  % Earth rate in the t-frame

% Second row:
    F21 = -vec2ss(C_t__b_hat * f_b__i_b_tilde); % Vector to Skew-Symmetric
  % Now build F23
    r_e__e_b_hat = r_e__e_t + C_e__t * r_t__t_b_hat;
    [L_b_hat, lambda_b_hat, h_b_hat] = xyz2llh(r_e__e_b_hat, P);
    gamma_e__i_b = gamma__i_b(r_e__e_b_hat, P);
    r_e__e_S = Geo_Radius(L_b_hat, P);
 
    F23 = -C_t__e * 2 * gamma_e__i_b * r_e__e_b_hat' / (r_e__e_S * norm(r_e__e_b_hat)) * C_e__t;
     
    F = [ -Ohm_t__i_e   ,  O3               , O3
           F21          , -2* Ohm_t__i_e    , F23
           O3           ,  I3               , O3];

%% Build the B matrix: See lecture 29 slide 7
    B = [O3         , C_t__b_hat
         C_t__b_hat , O3
         O3         , O3];

%% Transform Eqns from continuous-time to discrete-time: Lecture 30 slides 9-10
    Phi = eye(9) + F*dt;                % Estimate of exp(F dt) = I + F dt + F^2 dt^2 /2! + ...
	G  = (eye(9)*dt + F*dt^2/2) * B;    % Estimate of G = A^-1 (exp(F dt) - I ) B = (I dt + F dt^2 /2! + ...) B

    Delta_PVAk = Phi*Delta_PVAk_1 + G * [Df_b__i_b; Dw_b__i_b];

    Delta_PVAk_1 = Delta_PVAk;          % Store Delta_PVA(k) into Delta_PVA(k-1) for next iteration
end

Dk_t__bk = Delta_PVAk(1:3,1);   % Extract the Attitude errror terms
[y, p, r] = dcm2ypr(k2dcm(Dk_t__bk));
Dpsi_t__bk = [r; p; y];
Dv_t__t_bk = Delta_PVAk(4:6,1);   % Extract the velocity errror terms
Dr_t__t_bk = Delta_PVAk(7:9,1);   % Extract the position errror terms
end     % End of function

== matlab function qbot2_sim_2019b/Odometry Stage 1/MATLAB Function ==
  data: w_t__t_b_odo output; v_l input; v_b__t_b_odo output; v_r input; P parameter
%% Odometry Mechanization
function [w_t__t_b_odo, v_b__t_b_odo]= odo_mech(v_l, v_r, P)
                                                     
% Return Angular Velocity
w_t__t_b_odo = [0; 0; (v_l - v_r)/(2*P.radius)];

% Return Speed
v_b__t_b_odo = [((v_l + v_r)/2); 0; 0];

== matlab function qbot2_sim_2019b/IMU Error Reconciliation/IMU Error Reconciliation ==
  data: r_t__t_b_meas input; r_t__t_b_est output; v_t__t_b_meas input; C_t__b_meas input; v_t__t_b_est output; C_t__b_est output; delta_r_t__t_b_est input; delta_v_t__t_b_est input; delta_C_t__b_est input; P parameter
function [r_t__t_b_est, v_t__t_b_est, C_t__b_est] = ...
    imu_error_reconcile(r_t__t_b_meas, v_t__t_b_meas, C_t__b_meas, ...
                        delta_r_t__t_b_est, delta_v_t__t_b_est, delta_C_t__b_est, P)

                    
% No reconciliation for pure imu only
if (P.aiding_sensor_config == 0)
    
    r_t__t_b_est = r_t__t_b_meas;
    v_t__t_b_est = v_t__t_b_meas;
    C_t__b_est = C_t__b_meas;
    
    if (P.use_barometer == true)
        r_t__t_b_est(3) = r_t__t_b_meas(3) - delta_r_t__t_b_est(3);
    end


% Adjust for every other aiding sensor config
else
                    
    % Reconclie Position
    r_t__t_b_est = r_t__t_b_meas - delta_r_t__t_b_est;
    
    % Reconcile Velocity
    v_t__t_b_est = v_t__t_b_meas - delta_v_t__t_b_est;
    
    % Reconclie Attitude
    C_t__b_est = C_t__b_meas * delta_C_t__b_est;

end
